simulink model "untitled"  (R2014a)
settings: Solver=ode3  StartTime=0.0  StopTime=30  RelTol=1e-3
libraries: arduino_io_lib x5, simulink x2
settings Model: Creator=omar_  LastModifiedBy=omar_
settings SolverCC: AutoInsertRateTranBlk=on

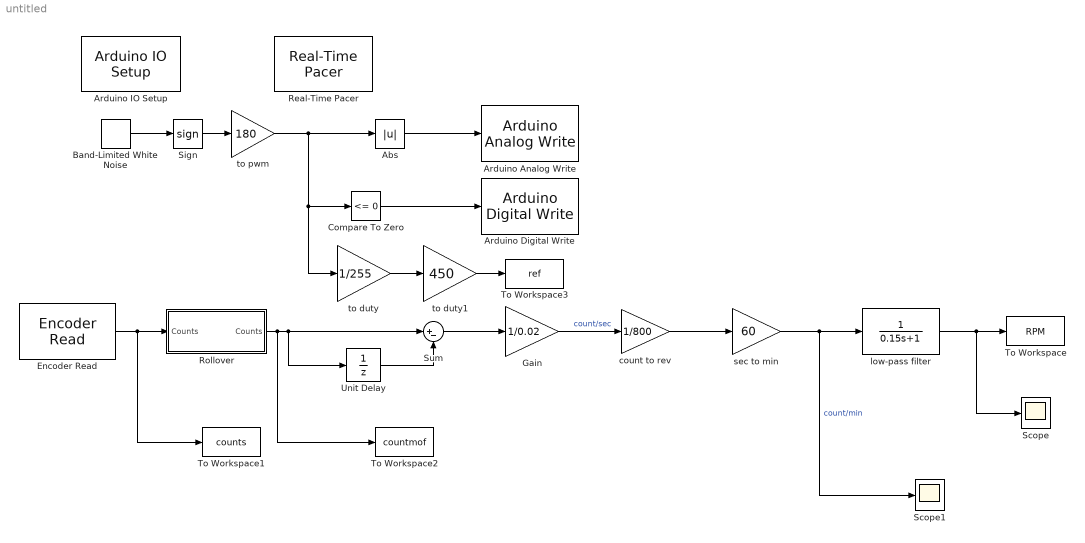
== system untitled ==
  Abs : Abs  OutDataTypeStr=uint16
  Arduino Analog Write : arduino_io_lib/Arduino Analog Write  arduinoVar=Temporary arduino variable: Arduino1  arduinoPin=5  T=0.2
  Arduino Digital Write : arduino_io_lib/Arduino Digital Write  arduinoVar=Temporary arduino variable: Arduino1  arduinoPin=6  T=0.2
  Arduino IO Setup : arduino_io_lib/Arduino IO Setup  Priority=3  arduinoVar=Temporary arduino variable: Arduino1  workspaceVarName=a  comPort=COM12
  Band-Limited White Noise : simulink/Sources/Band-Limited White Noise  Cov=[0.1]  Ts=3  seed=[23341]
  Compare To Zero : simulink/Logic and Bit Operations/Compare To Zero  relop=<=  OutDataTypeStr=boolean
  Encoder Read : arduino_io_lib/Encoder Read  arduinoVar=Temporary arduino variable: Arduino1  encNum=1  pinA=21  pinB=20  DbDl=0  T=0.02
  Gain : Gain  Gain=1/0.02
  Real-Time Pacer : arduino_io_lib/Real-Time Pacer  simTimePerRealTime=1
  Rollover : Subsystem
  Scope : Scope
      settings: TimeRange=20  YMin=280  YMax=380  Decimation=3
  Scope1 : Scope
      settings: TimeRange=30  YMin=-800  YMax=800  Decimation=3
  Sign : Signum
  Sum : Sum  Inputs=|+-
  To Workspace : ToWorkspace  VariableName=RPM  SampleTime=-1
  To Workspace1 : ToWorkspace  VariableName=counts  SampleTime=-1
      settings: Save2DSignal=2-D array (concatenate along first dimension)
  To Workspace2 : ToWorkspace  VariableName=countmof  SampleTime=-1
      settings: Save2DSignal=2-D array (concatenate along first dimension)
  To Workspace3 : ToWorkspace  VariableName=ref  SampleTime=0.02
  Unit Delay : UnitDelay  SampleTime=-1
  count to rev : Gain  Gain=1/800
  low-pass filter : TransferFcn  Denominator=[0.15 1]
  sec to min : Gain  Gain=60
  to duty : Gain  Gain=1/255
  to duty1 : Gain  Gain=450
  to pwm : Gain  Gain=180
  wires:
  Unit Delay/1 -> Sum/2
  Sum/1 -> Gain/1
  low-pass filter/1 -> Scope/1, To Workspace/1
  Encoder Read/1 -> To Workspace1/1, Rollover/1(Counts)
  Band-Limited White Noise/1 -> Sign/1
  Sign/1 -> to pwm/1
  to duty1/1 -> To Workspace3/1
  to duty/1 -> to duty1/1
  Rollover/1("Counts ") -> To Workspace2/1, Unit Delay/1, Sum/1
  Abs/1 -> Arduino Analog Write/1
  Compare To Zero/1 -> Arduino Digital Write/1
  Gain/1 -> count to rev/1  "count/sec"
  count to rev/1 -> sec to min/1
  sec to min/1 -> Scope1/1, low-pass filter/1  "count/min"
  to pwm/1 -> Abs/1, Compare To Zero/1, to duty/1

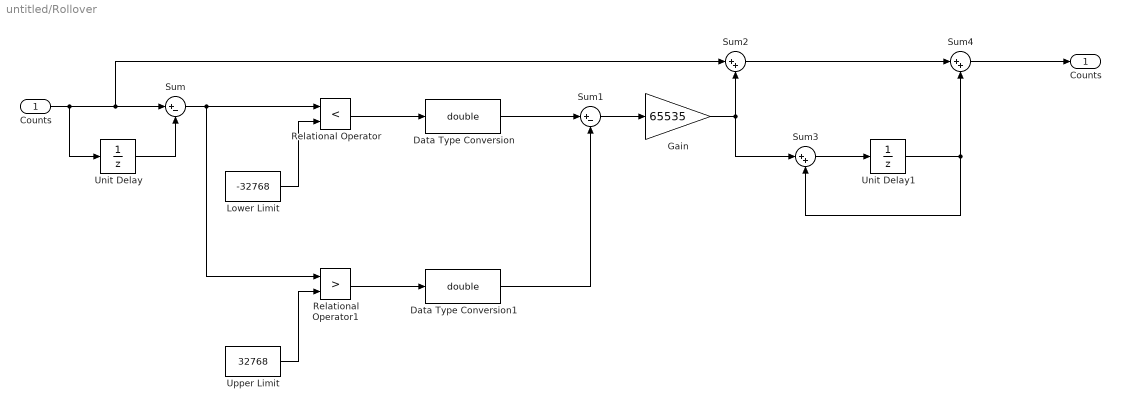
== system untitled/Rollover ==
  Counts : Inport
  Data Type Conversion : DataTypeConversion  OutDataTypeStr=double  RndMeth=Zero
  Data Type Conversion1 : DataTypeConversion  OutDataTypeStr=double  RndMeth=Zero
  Gain : Gain  Gain=65535
  Lower Limit : Constant  Value=-32768
  Relational Operator : RelationalOperator  Operator=<  OutDataTypeStr=boolean
  Relational Operator1 : RelationalOperator  Operator=>  OutDataTypeStr=boolean
  Sum : Sum  Inputs=|+-
  Sum1 : Sum  Inputs=|+-
  Sum2 : Sum  Inputs=|++
  Sum3 : Sum  Inputs=|++
  Sum4 : Sum  Inputs=|++
  Unit Delay : UnitDelay  SampleTime=-1
  Unit Delay1 : UnitDelay  SampleTime=-1
  Upper Limit : Constant  Value=32768
  "Counts " : Outport
  wires:
  Counts/1 -> Unit Delay/1, Sum2/1, Sum/1
  Unit Delay/1 -> Sum/2
  Sum/1 -> Relational Operator/1, Relational Operator1/1
  Lower Limit/1 -> Relational Operator/2
  Upper Limit/1 -> Relational Operator1/2
  Relational Operator/1 -> Data Type Conversion/1
  Relational Operator1/1 -> Data Type Conversion1/1
  Data Type Conversion1/1 -> Sum1/2
  Data Type Conversion/1 -> Sum1/1
  Sum1/1 -> Gain/1
  Gain/1 -> Sum3/1, Sum2/2
  Sum4/1 -> "Counts "/1
  Sum2/1 -> Sum4/1
  Sum3/1 -> Unit Delay1/1
  Unit Delay1/1 -> Sum4/2, Sum3/2
